simulink model "controlled_rectifier"  (R2023b)
settings: Solver=ode23tb  StartTime=0.0  StopTime=0.08  MaxStep=1e-4  RelTol=1e-3  EnableMultiTasking=on
InitFcn:
  | V=311.12
  | F=50
  | R=0.5
  | IO=10
  | VO=135
  | A=1
  | P=50
  | PA=0.02
  | AN1=(30*0.02)/360
  | AN2=(210*0.02)/360
libraries: spsThyristorLib x4, spsVoltageMeasurementLib x4, spsCurrentMeasurementLib x2, spsFourierLib x2, spsRMSLib x2, spsACVoltageSourceLib x1, spsDCVoltageSourceLib x1, spsControlledCurrentSourceLib x1, spsSeriesRLCBranchLib x1, spspowerguiLib x1
settings Model: Creator=s18elme05  LastModifiedBy=dhana
settings SolverCC: AlgebraicLoopSolver=TrustRegion
settings DataIOCC: LimitDataPoints=on  SaveFormat=Array  ReturnWorkspaceOutputs=off
settings OptimizationCC: ExpressionDepthLimit=2147483647  InitFltsAndDblsToZero=on  LifeSpan=inf
settings DebuggingCC: UnderspecifiedInitializationDetection=Classic  MergeDetectMultiDrivingBlocksExec=none  SolverPrmCheckMsg=warning  FcnCallInpInsideContextMsg=warning  UnconnectedInputMsg=warning  UnconnectedOutputMsg=warning  UnconnectedLineMsg=warning  StateNameClashWarn=warning  SFUnexpectedBacktrackingDiag=warning  SFNoUnconditionalDefaultTransitionDiag=warning  SFExecutionAtInitializationDiag=none  ArithmeticOperatorsInVariantConditions=warning
settings HardwareCC: ProdBitPerPointer=32  ProdBitPerSizeT=32  ProdBitPerPtrDiffT=32  ProdLargestAtomicFloat=None  ProdIntDivRoundTo=Undefined  ProdEndianess=Unspecified  ProdWordSize=32  ProdHWDeviceType=32-bit Generic
settings ModelReferenceCC: EnableRefExpFcnMdlSchedulingChecks=on  PropagateSignalLabelsOutOfModel=off
settings SFSimCC: SimUseLocalCustomCode=off  CustomCodeUndefinedFunction=UseInterfaceOnly
settings RTWCC: RTWUseLocalCustomCode=off
settings CodeAppCC: StateflowObjectComments=on
settings GRTTargetCC: TargetLangStandard=C89/C90 (ANSI)  CombineOutputUpdateFcns=off  GRTInterface=on
settings ConfigComp: CovMetricSettings=dw  CovSaveCumulativeToWorkspaceVar=on  CovSaveSingleToWorkspaceVar=on  CovExternalEMLEnable=off
settings SimscapeCC: SimscapeNormalizeSystem=off

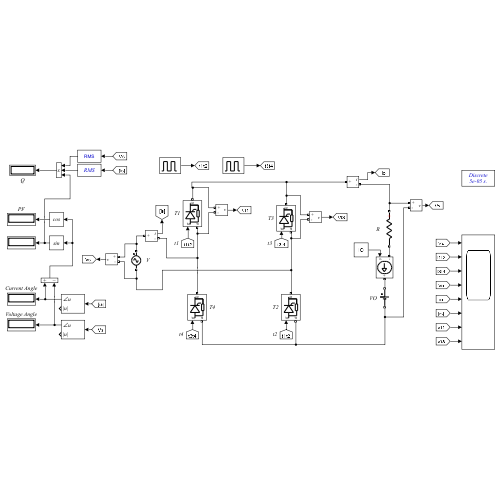
[thumbnail: Simulink's stored preview of the top-level diagram]
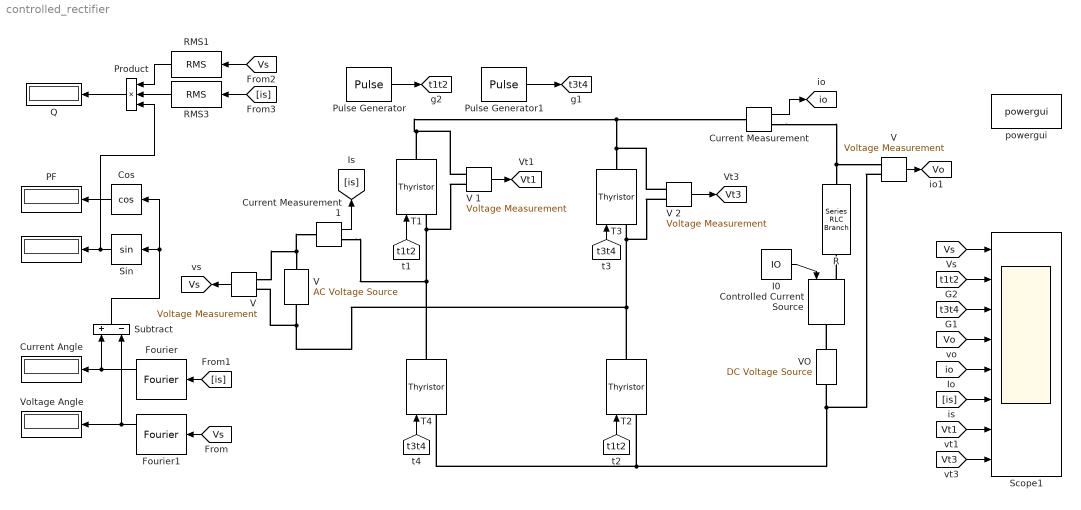
== system controlled_rectifier ==
  "  " : Display
  " V" : spsACVoltageSourceLib/AC Voltage Source  Amplitude=V  Phase=0  Frequency=F  SampleTime=0  Measurements=None  BusType=swing  Pref=10e3  Qref=0  Qmin=-inf  Qmax=+inf
  " VO" : spsDCVoltageSourceLib/DC Voltage Source  Amplitude=VO  Measurements=None
  Controlled Current Source : spsControlledCurrentSourceLib/Controlled Current Source  Initialize=on  Source_Type=AC  Amplitude=0  Phase=0  Frequency=0  Measurements=None
  Cos : Trigonometry  Operator=cos
  Current Angle : Display
  Current Measurement : spsCurrentMeasurementLib/Current Measurement  PhasorSimulation=off  OutputType=Complex  PSBequivalent=0
  Current Measurement1 : spsCurrentMeasurementLib/Current Measurement  PhasorSimulation=off  OutputType=Complex  PSBequivalent=0
  Fourier : spsFourierLib/Fourier  Freq=50  n=1  InInit=[0, 0]  Ts=0
  Fourier1 : spsFourierLib/Fourier  Freq=50  n=1  InInit=[0, 0]  Ts=0
  I0 : Constant  Value=IO
  PF : Display
  Product : Product  Inputs=3
  Pulse Generator : DiscretePulseGenerator  PulseType=Time based  Amplitude=A  Period=PA  PulseWidth=P  PhaseDelay=AN1
  Pulse Generator1 : DiscretePulseGenerator  PulseType=Time based  Amplitude=A  Period=PA  PulseWidth=P  PhaseDelay=AN2
  Q : Display
  R : spsSeriesRLCBranchLib/Series RLC Branch  LConnTagsString=__new0  RConnTagsString=__new0  BranchType=R  Resistance=R  Inductance=1e-3  SetiL0=off  InitialCurrent=0  Capacitance=1e-6  Setx0=off  InitialVoltage=0  Measurements=None
  RMS1 : spsRMSLib/RMS  TrueRMS=on  Freq=50  RMSInit=120  Ts=0
  RMS3 : spsRMSLib/RMS  TrueRMS=on  Freq=50  RMSInit=120  Ts=0
  Scope1 : Scope  NumInputPorts=8
  Sin : Trigonometry
  Subtract : Sum  Inputs=+-
  T{1..4} (4 alike) : spsThyristorLib/Thyristor  Ron=0.001  Lon=0  Vf=0.8  IC=0  Rs=500  Cs=250e-9  Measurements=off
  V : spsVoltageMeasurementLib/Voltage Measurement  PhasorSimulation=off  OutputType=Complex  PSBequivalent=0
  "V " : spsVoltageMeasurementLib/Voltage Measurement  PhasorSimulation=off  OutputType=Complex  PSBequivalent=0
  V 1 : spsVoltageMeasurementLib/Voltage Measurement  PhasorSimulation=off  OutputType=Complex  PSBequivalent=0
  V 2 : spsVoltageMeasurementLib/Voltage Measurement  PhasorSimulation=off  OutputType=Complex  PSBequivalent=0
  Voltage Angle : Display
  powergui : spspowerguiLib/powergui  SimulationMode=Discrete  SampleTime=50e-6  frequency=60  Iterations=50  frequencyindice=0  Pbase=100e6  ErrMax=1e-4  UnitsV=kV  UnitsW=MW  buscounter=0  FunctionMessages=off  echomessages=off  EnableUseOfTLC=off  CurrentSourceSwitches=off  DisableSnubberDevices=off  DisableRonSwitches=off  DisableVfSwitches=off  DisplayEquations=off  AutomaticDiscreteSolvers=off  SolverType=Tustin/Backward Euler (TBE)  Interpol=off  ExternalGateDelay=off  methode=off  Ts=0  x0status=blocks  SPID=off  SwTol=0  HookPort=off  NonlinearTolerance=1e-4  nMaxIteration=100  ContinueOnMaxIteration=off  RestoreLinks=warning  ResistiveCurrentMeasurement=off  Frange=[0:2:500]  Ylog=off  Xlog=on  ShowGrid=off  save=off  variable=ZData  structure=aa  ZoomFFT=on  StartTime=0.06  cycles=3  DisplayStyle=1  fundamental=50  FreqAxis=on  MaxFrequency=1000  frequencyindicesteady=1  RmsSteady=1  display=off
  tag scope: Vo=global, Vs=global, Vt1=global, Vt3=global, io=global, t1t2=global, t3t4=global
  wires:
  I0/1 -> Controlled Current Source/1
  Current Measurement1/1 -> [is]
  V/1 -> [Vs]
  [Vs] -> Scope1/1
  V 1/1 -> [Vt1]
  V 2/1 -> [Vt3]
  Pulse Generator1/1 -> [t3t4]
  Current Measurement/1 -> [io]
  "V "/1 -> [Vo]
  [t3t4] -> T4/1
  [t3t4] -> T3/1
  Pulse Generator/1 -> [t1t2]
  [t1t2] -> T1/1
  [t1t2] -> T2/1
  [t1t2] -> Scope1/2
  [t3t4] -> Scope1/3
  [Vo] -> Scope1/4
  [io] -> Scope1/5
  [is] -> Scope1/6
  [Vt1] -> Scope1/7
  [Vt3] -> Scope1/8
  [Vs] -> Fourier1/1
  [is] -> Fourier/1
  Fourier1/2 -> Voltage Angle/1, Subtract/2
  Fourier/2 -> Current Angle/1, Subtract/1
  Subtract/1 -> Sin/1, Cos/1
  Cos/1 -> PF/1
  [is] -> RMS3/1
  [Vs] -> RMS1/1
  Product/1 -> Q/1
  Sin/1 -> Product/3, "  "/1
  RMS1/1 -> Product/1
  RMS3/1 -> Product/2
  connections:
  V/LConn2 -- " V"/LConn1 -- T2/RConn1 -- V 2/LConn2 -- T3/LConn1
  "V "/LConn2 -- T4/LConn1 -- T2/LConn1 -- " VO"/LConn1
  V/LConn1 -- Current Measurement1/LConn1 -- " V"/RConn1
  T1/RConn1 -- V 2/LConn1 -- T3/RConn1 -- Current Measurement/LConn1 -- V 1/LConn1
  Controlled Current Source/LConn1 -- R/RConn1
  Current Measurement/RConn1 -- R/LConn1 -- "V "/LConn1
  " VO"/RConn1 -- Controlled Current Source/RConn1
  T4/RConn1 -- Current Measurement1/RConn1 -- V 1/LConn2 -- T1/LConn1
